simulink model "rtwdemo_comments"  (Simulink 6.0)
settings: Solver=FixedStepDiscrete  SolverMode=SingleTasking  StartTime=0.0  StopTime=10.0  FixedStep=0.05  RelTol=1e-3
PreLoadFcn:
  | rtwdemo_comments_data;
values from neighbouring files (symbols this model uses):
  const_val = Simulink.Parameter    [rtwdemo_comments_data.m]
libraries: rtwdemowidgets x1, simulink x1
Description:
  | This model represents a mutual exclusion arbitrator.
  | If exactly one input is enabled, the output will be
  | its index; Otherwise, previous output will be used.
settings Model: Creator=The MathWorks Inc.  LastModifiedBy=batserve  ExtModeAutoUpdateStatusClock=off
settings DataIOCC: ExternalInput=[tim_var, data_var]  LoadExternalInput=on  SaveOutput=off  SaveTime=off
settings OptimizationCC: InlineParams=on  EnforceIntegerDowncast=off  StateBitsets=on  DataBitsets=on  UseTempVars=on  ZeroExternalMemoryAtStartup=off  ZeroInternalMemoryAtStartup=off  InitFltsAndDblsToZero=off  NoFixptDivByZeroProtection=on  OptimizeModelRefInitCode=on  LifeSpan=1
settings DebuggingCC: CheckExecutionContextPreStartOutputMsg=on  CheckExecutionContextRuntimeOutputMsg=on
settings RTWCC: SystemTargetFile=ert.tlc  TLCOptions=-p0 -aWarnNonSaturatedBlocks=0  GenCodeOnly=on  TemplateMakefile=ert_default_tmf  Description=RTW Embedded Coder (no auto configuration)  GenerateReport=on  RTWVerbose=off  ProcessScript=ert_make_rtw_hook  IncludeHyperlinkInReport=on  LaunchReport=on
settings CodeAppCC: ForceParamTrailComments=on  IgnoreCustomStorageClasses=off  SimulinkDataObjDesc=on  SFDataObjDesc=on  CustomSymbolStr=$N$M  CustomCommentsFcn=rtwdemo_comments_mptfun.m  InsertBlockDesc=on  EnableCustomComments=on
settings ERTTargetCC: TargetFcnLib=ansi_tfl_tmw.mat  GenFloatMathFcnCalls=ANSI_C  GenerateSampleERTMain=on  IncludeMdlTerminateFcn=off  SupportNonFinite=off  SupportComplex=off  SupportContinuousTime=on  SupportNonInlinedSFcns=on  InlinedParameterPlacement=NonHierarchical  RootIOFormat=Individual Arguments  ERTCustomFileTemplate=example_file_process.tlc  InitialValueSource=Model

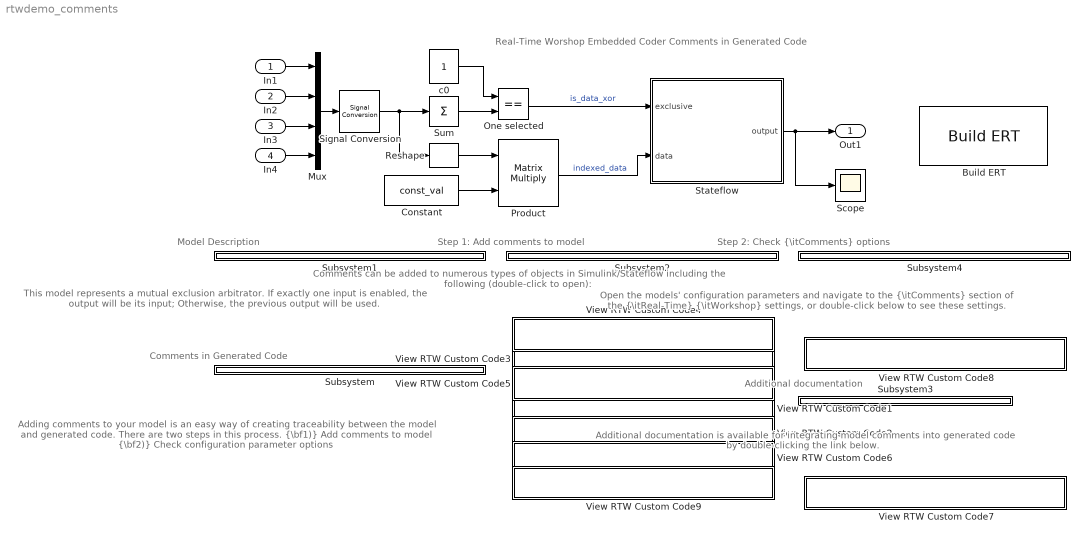
== system rtwdemo_comments ==
  note: This model represents a mutual exclusion
      | arbitrator.  If exactly one input is enabled,
      | the output will be its input; Otherwise,
      | the previous output will be used.
  note: Real-Time Worshop Embedded Coder
      | Comments in Generated Code
  note: Comments in Generated Code
  note: Adding comments to your model is an easy
      | way of creating traceability between the model
      | and generated code.  There are two steps in
      | this process.
      |
      |   {\bf1)} Add comments to model
      |   {\bf2)} Check configuration parameter options
  note: Additional documentation
  note: Additional documentation is available
      | for integrating model comments into
      | generated code by double-clicking the
      | link below.
  note: Comments can be added to numerous types
      | of objects in Simulink/Stateflow including the
      | following (double-click to open):
  note: Model Description
  note: Open the models' configuration parameters
      | and navigate to the {\itComments} section of
      | the {\itReal-Time} {\itWorkshop} settings, or
      | double-click below to see these settings.
  note: Step 1: Add comments to model
  note: Step 2: Check {\itComments} options
  In1 : Inport  Port=1  PortDimensions=1  DataType=double  LatchInput=off
  In2 : Inport  Port=2  PortDimensions=1  DataType=double  LatchInput=off
  In3 : Inport  Port=3  PortDimensions=1  DataType=double  LatchInput=off
  In4 : Inport  Port=4  PortDimensions=1  DataType=double  LatchInput=off
  Build ERT : rtwdemowidgets/Build ERT  attrib_overrides={}
  Constant : Constant  Value=const_val  VectorParams1D=off  OutDataTypeMode=double
  Mux : Mux
  "One selected " : RelationalOperator  Description=This block determines if exactly one input is enabled.  Operator===  LogicOutDataTypeMode=Boolean
  Product : Product  Description=This block determines the output index by taking the inner product of the vector of inputs and [1 2 3 4].  Multiplication=Matrix(*)  OutDataTypeMode=double  RndMeth=Zero
  Reshape : simulink/Math Operations/Reshape  OutputDimensionality=Row vector  OutputDimensions=[1,1]
  Scope : Scope
      settings: YMin=0.95  YMax=1.05
  Signal Conversion : SignalConversion  ConversionOutput=Contiguous copy  OverrideOpt=on
  Stateflow : Stateflow chart  Description=|  TreatAsAtomicUnit=on  PropExecContextAcrossSSBoundary=on
      | Stateflow block decides the index output by following logic   
      | 1. If one and only one input signal is enabled, the index will
      | refer to the enabled signal line.                             
      | 2. Otherwise, maintain the old value.
  Subsystem : Subsystem  PropExecContextAcrossSSBoundary=on
  Subsystem1 : Subsystem  PropExecContextAcrossSSBoundary=on
  Subsystem2 : Subsystem  PropExecContextAcrossSSBoundary=on
  Subsystem3 : Subsystem  PropExecContextAcrossSSBoundary=on
  Subsystem4 : Subsystem  PropExecContextAcrossSSBoundary=on
  Sum : Sum  Description=This block counts the number of enabled inputs.  Inputs=+  OutDataTypeMode=double  OutScaling=2^-10  InputSameDT=on
  View RTW Custom Code1 : Subsystem  PropExecContextAcrossSSBoundary=on
      mask init:
      | pos    = get_param(gcb, 'Position');
      | width  = pos(3) - pos(1);
      | height = pos(4) - pos(2);
      | 
      | 
      | % Compute arrow coordinates
      | arrowW = width  / 20;
      | arrowH = height / 2.5;
      | arrowX = width  / 50;
      | arrowY = height / 3;
      | arrowXvec = [arrowX, arrowX, arrowX + arrowW];
      | arrowYvec = [arrowY, arrowY + arrowH, arrowY + arrowH / 2];
      | 
      | % Compute text position
      | textXbuff = width / 30;
      | textX  = arrowX + arrowW + textXbuff;
      | textY  = height / 2;
      settings: OpenFcn=DAStudio.Dialog(is_data_xor);
      mask Display:
      | patch(arrowXvec, arrowYvec);
      | text(textX, textY, 'Simulink Signal Object');
  View RTW Custom Code2 : Subsystem  PropExecContextAcrossSSBoundary=on
      mask init: same as rtwdemo_comments/View RTW Custom Code1
      settings: OpenFcn=DAStudio.Dialog(const_val);
      mask Display:
      | patch(arrowXvec, arrowYvec);
      | text(textX, textY, 'Simulink Parameter Object');
  View RTW Custom Code3 : Subsystem  PropExecContextAcrossSSBoundary=on
      mask init: same as rtwdemo_comments/View RTW Custom Code1
      settings: OpenFcn=|
      | state=find(sfroot,'-isa','Stateflow.State','-and','Name','Normal');
      | sf('Open',state.id);
      | DAStudio.Dialog(state);
      mask Display:
      | patch(arrowXvec, arrowYvec);
      | text(textX, textY, 'Stateflow State');
  View RTW Custom Code4 : Subsystem  PropExecContextAcrossSSBoundary=on
      mask init: same as rtwdemo_comments/View RTW Custom Code1
      settings: OpenFcn=|
      | block=[bdroot, '/Product'];
      | hilite_system(block);
      | open_system(block, 'property');
      mask Display:
      | patch(arrowXvec, arrowYvec);
      | text(textX, textY, 'Simulink Block');
  View RTW Custom Code5 : Subsystem  PropExecContextAcrossSSBoundary=on
      mask init: same as rtwdemo_comments/View RTW Custom Code1
      settings: OpenFcn=|
      | trans=find(sfroot,'-isa','Stateflow.Transition','-and','LabelString','// After initialize');
      | sf('Open',trans.id);
      | DAStudio.Dialog(trans);
      mask Display:
      | patch(arrowXvec, arrowYvec);
      | text(textX, textY, 'Stateflow Transition');
  View RTW Custom Code6 : Subsystem  PropExecContextAcrossSSBoundary=on
      mask init: same as rtwdemo_comments/View RTW Custom Code1
      settings: OpenFcn=DAStudio.Dialog(indexed_data);
      mask Display:
      | patch(arrowXvec, arrowYvec);
      | text(textX, textY, 'MPT Signal Object');
  View RTW Custom Code7 : Subsystem  PropExecContextAcrossSSBoundary=on
      mask init: same as rtwdemo_comments/View RTW Custom Code1
      settings: OpenFcn=helpview([docroot '/mapfiles/ecoder_ug.map'], 'ecoder_comments_pane')
      mask Display:
      | patch(arrowXvec, arrowYvec);
      | text(textX, textY, 'Comments Documentation');
  View RTW Custom Code8 : Subsystem  PropExecContextAcrossSSBoundary=on
      mask init: same as rtwdemo_comments/View RTW Custom Code1
      settings: OpenFcn=|
      | model = bdroot;
      | slCfgPrmDlg(model,'Open');
      | slCfgPrmDlg(bdroot,'TurnToPage','Comments');
      mask Display:
      | patch(arrowXvec, arrowYvec);
      | text(textX, textY, 'Open Comments Settings');
  View RTW Custom Code9 : Subsystem  PropExecContextAcrossSSBoundary=on
      mask init: same as rtwdemo_comments/View RTW Custom Code1
      settings: OpenFcn=edit rtwdemo_comments_mptfun.m;
      mask Display:
      | patch(arrowXvec, arrowYvec);
      | text(textX, textY, 'MPT Callback Function');
  c0 : Constant
  Out1 : Outport
  wires:
  Mux/1 -> Signal Conversion/1
  Constant/1 -> Product/2
  c0/1 -> "One selected "/1
  Sum/1 -> "One selected "/2
  "One selected "/1 -> Stateflow/1(exclusive)  "is_data_xor"
  Product/1 -> Stateflow/2(data)  "indexed_data"
  Stateflow/1(output) -> Out1/1, Scope/1
  In1/1 -> Mux/1
  In2/1 -> Mux/2
  In3/1 -> Mux/3
  In4/1 -> Mux/4
  Signal Conversion/1 -> Sum/1, Reshape/1
  Reshape/1 -> Product/1

== system rtwdemo_comments/Subsystem ==

== system rtwdemo_comments/Subsystem1 ==

== system rtwdemo_comments/Subsystem2 ==

== system rtwdemo_comments/Subsystem3 ==

== system rtwdemo_comments/Subsystem4 ==

== system rtwdemo_comments/View RTW Custom Code1 ==

== system rtwdemo_comments/View RTW Custom Code2 ==

== system rtwdemo_comments/View RTW Custom Code3 ==

== system rtwdemo_comments/View RTW Custom Code4 ==

== system rtwdemo_comments/View RTW Custom Code5 ==

== system rtwdemo_comments/View RTW Custom Code6 ==

== system rtwdemo_comments/View RTW Custom Code7 ==

== system rtwdemo_comments/View RTW Custom Code8 ==

== system rtwdemo_comments/View RTW Custom Code9 ==

== stateflow chart Stateflow ==
  state Normal
    settings: description=This state determines the value of the output after the intialization.
    (default) -> (junction 5)
    (junction 5) -> (junction 6) : [exclusive]
      settings: description=This transition is taken when exactly one input is enabled.
    (junction 6) -> (junction 7) : {output=data;}
      settings: description=This transition assigns the output to the index of the only enabled input.
    (junction 7) -> (junction 8)
    (junction 5) -> (junction 8) : // Output has
        | // previous value
    Normal -> (junction 5)
  state First
    entry: output=1;
    settings: description=The state is activated at initialization.
  (default) -> First
  First -> Normal : // After initialize
    settings: description=After initialization, transfer to the normal state.
  data: exclusive input boolean; data input inherited; output output int32 size=1
